simulink model "questionario3"  (R2020a)
settings: Solver=VariableStepAuto  StartTime=0.0  StopTime=1000  RelTol=1e-3
libraries: simulink x2
settings Model: Creator=Gabriel  LastModifiedBy=Gabriel

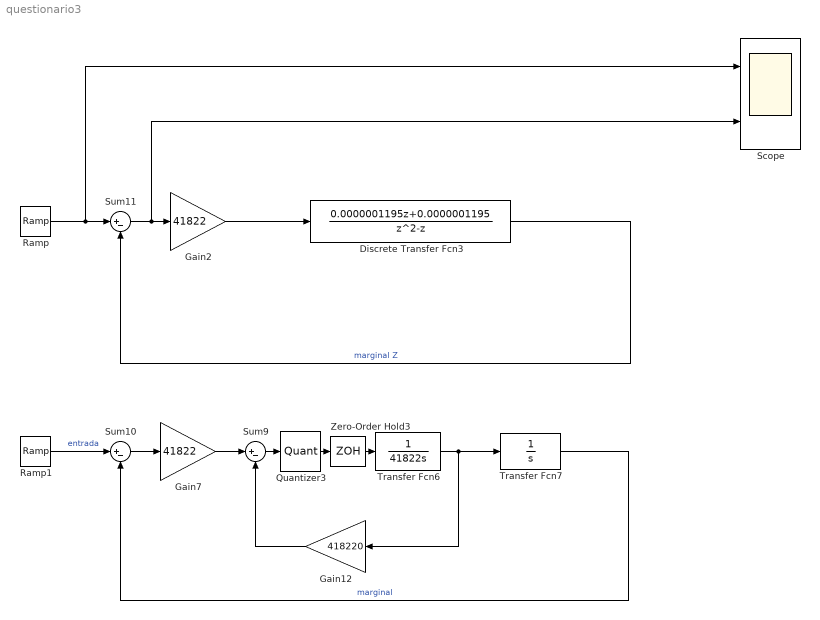
== system questionario3 ==
  Discrete Transfer Fcn3 : DiscreteTransferFcn  Numerator=[0.0000001195 0.0000001195]  Denominator=[1 -1 0]
  Gain12 : Gain  Gain=418220
  Gain2 : Gain  Gain=41822
  Gain7 : Gain  Gain=41822
  Quantizer3 : Quantizer  QuantizationInterval=0.1  LinearizeAsGain=off
  Ramp : simulink/Sources/Ramp  slope=1  start=0  InitialOutput=0
  Ramp1 : simulink/Sources/Ramp  slope=1  start=0  InitialOutput=0
  Scope : Scope  NumInputPorts=2
  Sum10 : Sum  Inputs=|+-
  Sum11 : Sum  Inputs=|+-
  Sum9 : Sum  Inputs=|+-
  Transfer Fcn6 : TransferFcn  Denominator=[41822 0]
  Transfer Fcn7 : TransferFcn  Denominator=[1 0]
  Zero-Order Hold3 : ZeroOrderHold  SampleTime=0.1
  wires:
  Gain12/1 -> Sum9/2
  Zero-Order Hold3/1 -> Transfer Fcn6/1
  Transfer Fcn6/1 -> Gain12/1, Transfer Fcn7/1
  Quantizer3/1 -> Zero-Order Hold3/1
  Sum9/1 -> Quantizer3/1
  Ramp/1 -> Scope/1, Sum11/1
  Gain2/1 -> Discrete Transfer Fcn3/1
  Gain7/1 -> Sum9/1
  Ramp1/1 -> Sum10/1  "entrada"
  Sum10/1 -> Gain7/1
  Sum11/1 -> Scope/2, Gain2/1
  Transfer Fcn7/1 -> Sum10/2  "marginal"
  Discrete Transfer Fcn3/1 -> Sum11/2  "marginal Z"
